simulink model "New_kinematic_viscosity"  (Simulink 8.2)
settings: Solver=FixedStepDiscrete  StartTime=0.0  StopTime=10  FixedStep=1  RelTol=1e-3
libraries: carnot x3
settings Model: Creator=awohlfei  LastModifiedBy=drhf
settings DebuggingCC: FcnCallInpInsideContextMsg=EnableAllAsWarning
settings GRTTargetCC: CombineOutputUpdateFcns=on  GRTInterface=off

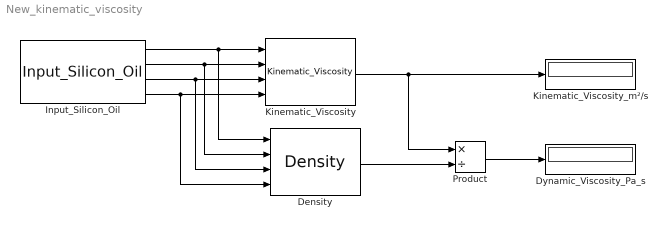
== system New_kinematic_viscosity ==
  Density : carnot/Basic/Material_Properties/Density  VariantControl=CarlibClassic  INPUTARGUMENTS=state variables (classic)  DEBUGLEVEL=DEBUGLEVEL  MAXTOTALWARNINGS=inf  MAXCONSECUTIVEWARNINGS=inf  WRITETOFILE=0  FILENAME='errors.txt'
  Dynamic_Viscosity_Pa_s : Display
  Input_Silicon_Oil : carnot/Basic/Material_Properties/Input_Silicon_Oil  T=50  p=1e5
  Kinematic_Viscosity : carnot/Basic/Material_Properties/Kinematic_Viscosity  VariantControl=CarlibClassic  INPUTARGUMENTS=state variables (classic)  DEBUGLEVEL=WARNINGLEVEL  MAXTOTALMESSAGES=inf  MAXCONSECUTIVEMESSAGES=inf  WRITETOFILE=0  FILENAME='errors.txt'
  Kinematic_Viscosity_m²/s : Display
  Product : Product  Inputs=*/
  wires:
  Kinematic_Viscosity/1 -> Product/1, Kinematic_Viscosity_m²/s/1
  Input_Silicon_Oil/1 -> Kinematic_Viscosity/1, Density/1
  Input_Silicon_Oil/2 -> Kinematic_Viscosity/2, Density/2
  Input_Silicon_Oil/4 -> Kinematic_Viscosity/4, Density/4
  Input_Silicon_Oil/3 -> Kinematic_Viscosity/3, Density/3
  Density/1 -> Product/2
  Product/1 -> Dynamic_Viscosity_Pa_s/1
